simulink model "sim_single_lin"  (R2018a)
settings: Solver=ode3  StartTime=0.0  StopTime=params.tf  FixedStep=1e-3  RelTol=1e-3
values from neighbouring files (symbols this model uses):
  A = sys.lin_sys.continuous.systems{1}.ss.a    [load_sys.m]
  B = sys.lin_sys.continuous.systems{1}.ss.b    [load_sys.m]
  C = dsys.c    [load_sys.m]
  Gamma = dsys.b    [load_sys.m]
  Ki = -K(:, n+1:end)    [load_control.m]
  Kp = K(:, 1:n)    [load_control.m]
  L = dlqe(Phi, Psi, C, Rw, Rv)    [load_control.m]
  params = catstruct(params, sys.params_str)    [run_sim.m]
  Phi = dsys.a    [load_sys.m]
  Psi = [zeros(2, 1); ones(2, 1)]    [load_control.m]
  Ts = dsys.ts    [load_sys.m]
  xhat0 = params.xhat0    [load_control.m]
settings Model: Creator=BPeixoto  LastModifiedBy=brunolnetto
settings DataIOCC: LimitDataPoints=on  SaveFormat=Array
settings OptimizationCC: BlockReduction=off  BooleanDataType=off  LifeSpan=inf
settings DebuggingCC: SaveWithParameterizedLinksMsg=none  UnderspecifiedInitializationDetection=Classic  MergeDetectMultiDrivingBlocksExec=none  SignalResolutionControl=TryResolveAllWithWarning  SFUnexpectedBacktrackingDiag=warning  SFNoUnconditionalDefaultTransitionDiag=warning  SFExecutionAtInitializationDiag=none
settings HardwareCC: ProdBitPerPointer=32  ProdBitPerSizeT=32  ProdBitPerPtrDiffT=32  ProdLargestAtomicFloat=None  ProdIntDivRoundTo=Undefined  ProdEndianess=Unspecified  ProdWordSize=32  ProdHWDeviceType=32-bit Generic  TargetUnknown=on
settings ModelReferenceCC: PropagateSignalLabelsOutOfModel=off
settings CodeAppCC: StateflowObjectComments=on
settings GRTTargetCC: TargetLangStandard=C89/C90 (ANSI)  GeneratePreprocessorConditionals=Disable all
settings ConfigComp: CovMetricSettings=dw  CovHtmlReporting=on  CovSaveCumulativeToWorkspaceVar=on  CovSaveSingleToWorkspaceVar=on  CovExternalEMLEnable=off  CovSFcnEnable=off

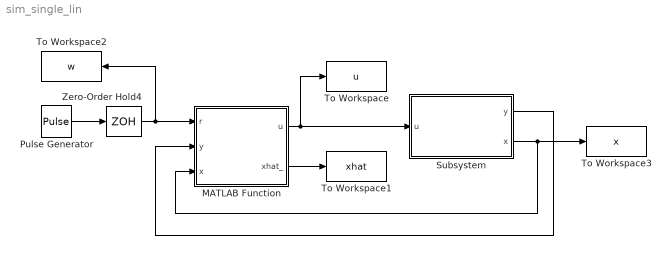
== system sim_single_lin ==
  MATLAB Function : MATLAB Function  TreatAsAtomicUnit=on
  Pulse Generator : DiscretePulseGenerator  PulseType=Time based  Amplitude=params.step_amplitude  Period=10  PulseWidth=50
  Subsystem : Subsystem
  To Workspace : ToWorkspace  VariableName=u  SaveFormat=Structure With Time  SampleTime=-1
  To Workspace1 : ToWorkspace  VariableName=xhat  SaveFormat=Structure With Time  SampleTime=Ts
  To Workspace2 : ToWorkspace  VariableName=w  SaveFormat=Structure With Time  SampleTime=Ts
  To Workspace3 : ToWorkspace  VariableName=x  SaveFormat=Structure With Time  SampleTime=-1
  Zero-Order Hold4 : ZeroOrderHold  SampleTime=Ts
  wires:
  Pulse Generator/1 -> Zero-Order Hold4/1
  Zero-Order Hold4/1 -> MATLAB Function/1(r), To Workspace2/1
  Subsystem/1(y) -> MATLAB Function/2(y)
  MATLAB Function/2(xhat_) -> To Workspace1/1
  MATLAB Function/1(u) -> To Workspace/1, Subsystem/1(u)
  Subsystem/2(x) -> To Workspace3/1, MATLAB Function/3(x)

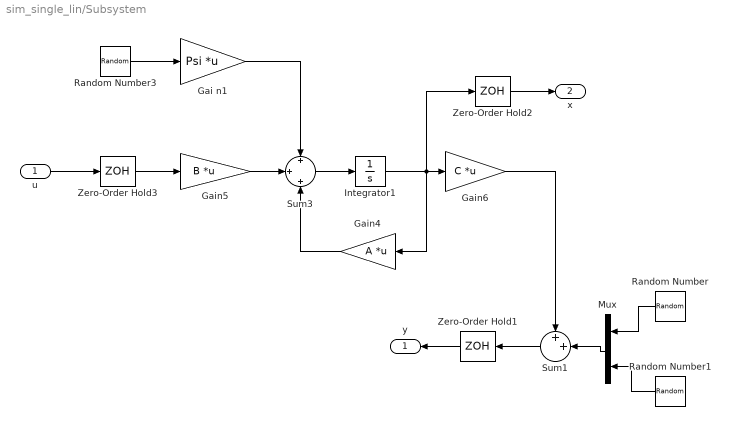
== system sim_single_lin/Subsystem ==
  u : Inport
  Gai n1 : Gain  Gain=Psi  Multiplication=Matrix(K*u) (u vector)
  Gain4 : Gain  Gain=A  Multiplication=Matrix(K*u) (u vector)
  Gain5 : Gain  Gain=B  Multiplication=Matrix(K*u) (u vector)
  Gain6 : Gain  Gain=C  Multiplication=Matrix(K*u) (u vector)
  Integrator1 : Integrator  InitialCondition=[params.q0,params.qp0 ] - params.x0
  Mux : Mux  Inputs=2
  Random Number : RandomNumber  Variance=params.Rv  SampleTime=Ts
  Random Number1 : RandomNumber  Variance=params.Rv  SampleTime=Ts
  Random Number3 : RandomNumber  Variance=params.Rw  SampleTime=Ts
  Sum1 : Sum  Inputs=++|
  Sum3 : Sum  Inputs=+|+|+
  Zero-Order Hold1 : ZeroOrderHold  SampleTime=Ts
  Zero-Order Hold2 : ZeroOrderHold  SampleTime=Ts
  Zero-Order Hold3 : ZeroOrderHold  SampleTime=Ts
  y : Outport
  x : Outport  Port=2
  wires:
  Random Number/1 -> Mux/1
  Gain5/1 -> Sum3/2
  Sum1/1 -> Zero-Order Hold1/1
  Sum3/1 -> Integrator1/1
  Zero-Order Hold3/1 -> Gain5/1
  Mux/1 -> Sum1/2
  Random Number1/1 -> Mux/2
  Gai n1/1 -> Sum3/1
  Zero-Order Hold1/1 -> y/1
  Gain4/1 -> Sum3/3
  Random Number3/1 -> Gai n1/1
  u/1 -> Zero-Order Hold3/1
  Zero-Order Hold2/1 -> x/1
  Integrator1/1 -> Zero-Order Hold2/1, Gain4/1, Gain6/1
  Gain6/1 -> Sum1/1

== matlab function sim_single_lin/MATLAB Function ==
  data: r input; u output; xhat_ output; y input; x input; Phi parameter; C parameter; L parameter; Gamma parameter; Kp parameter; Ki parameter; xhat0 parameter
function [u, xhat_] = controle(r, y, x, Phi, C, L, Gamma, Kp, Ki, xhat0)
    persistent v;
    persistent xhat;
    
    if(isempty(v))
        v = 0;
    end
        
    if(isempty(xhat))
        xhat = xhat0;
    end
        
    xhat_ = xhat;
    u = -Kp*xhat + Ki*v;
    v = v + r - y(1);
    
    xhat = Phi*xhat + Gamma*u + L*(y - C*xhat);
end
